simulink model "SMC"  (R2018a)
settings: Solver=VariableStepAuto  StartTime=0.0  StopTime=10.0  RelTol=1e-3
settings Model: Creator=R-YDL  LastModifiedBy=R-YDL

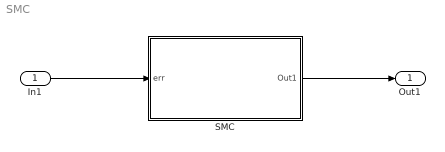
== system SMC ==
  In1 : Inport
  SMC : Subsystem  mask{C=0, e=0, K=0, A=0}
  Out1 : Outport
  wires:
  In1/1 -> SMC/1(err)
  SMC/1(Out1) -> Out1/1

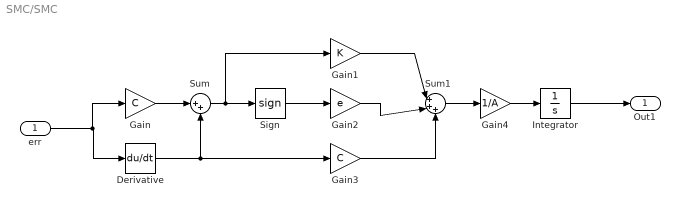
== system SMC/SMC ==
  err : Inport
  Derivative : Derivative
  Gain : Gain  Gain=C
  Gain1 : Gain  Gain=K
  Gain2 : Gain  Gain=e
  Gain3 : Gain  Gain=C
  Gain4 : Gain  Gain=1/A
  Integrator : Integrator
  Sign : Signum
  Sum : Sum  Inputs=|++
  Sum1 : Sum  Inputs=|+++
  Out1 : Outport
  wires:
  Integrator/1 -> Out1/1
  Sign/1 -> Gain2/1
  Gain1/1 -> Sum1/1
  Derivative/1 -> Gain3/1, Sum/2
  Gain3/1 -> Sum1/3
  Sum1/1 -> Gain4/1
  Gain/1 -> Sum/1
  Sum/1 -> Gain1/1, Sign/1
  err/1 -> Gain/1, Derivative/1
  Gain2/1 -> Sum1/2
  Gain4/1 -> Integrator/1
